simulink model "PLL"  (R2016a)
settings: Solver=ode45  StartTime=0.0  StopTime=stop  MaxStep=1e-6  RelTol=1e-3
values from neighbouring files (symbols this model uses):
  f = 9000    [Aufgabe5.m]
  K0 = 2*pi*400    (= 2513.27412287)    [Aufgabe5.m]
  tau1 = K0*Kd/w0^2    (= 0.000881744837074)    [Aufgabe5.m]
  tau2 = 2*zeta/w0-1/(K0*Kd)    (= 0.000376945917849)    [Aufgabe5.m]
libraries: dspvision x2, dsparch4 x1, commsynccomp2 x1
settings Model: Creator=Martin Buchholz  LastModifiedBy=Marcel
settings DataIOCC: LimitDataPoints=on  SaveFormat=Array  SignalLoggingSaveFormat=ModelDataLogs
settings OptimizationCC: ExpressionDepthLimit=2147483647
settings DebuggingCC: UnderspecifiedInitializationDetection=Classic  MergeDetectMultiDrivingBlocksExec=none  SolverPrmCheckMsg=warning  FcnCallInpInsideContextMsg=UseLocalSettings  StateNameClashWarn=warning
settings HardwareCC: ProdBitPerPointer=32  ProdLargestAtomicFloat=None  ProdIntDivRoundTo=Undefined  ProdEndianess=Unspecified  ProdWordSize=32  ProdHWDeviceType=32-bit Generic
settings ModelReferenceCC: PropagateSignalLabelsOutOfModel=off
settings GRTTargetCC: GeneratePreprocessorConditionals=Use local settings  CombineOutputUpdateFcns=off  GRTInterface=on
settings ConfigComp: CovModelRefEnable=Off

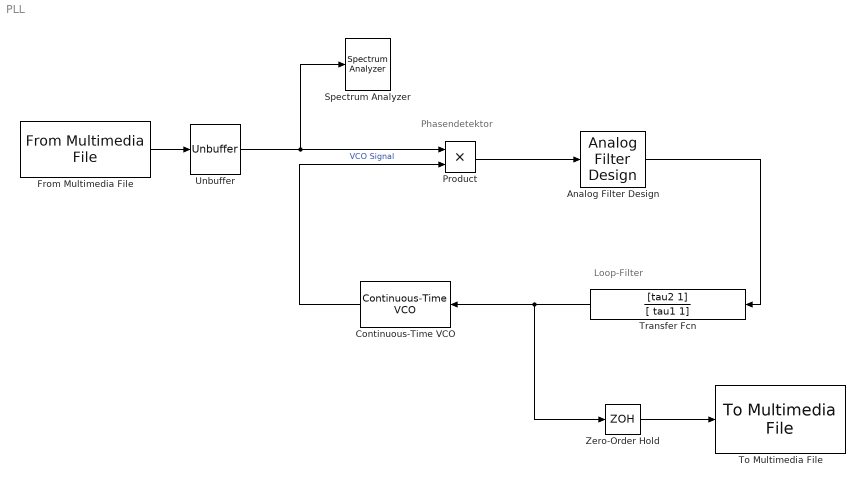
== system PLL ==
  note: Phasendetektor
  note: Loop-Filter
  Analog Filter Design : dsparch4/Analog Filter Design  method=Elliptic  filttype=Lowpass  N=4  Wlo=2*pi*f  Whi=80  Rp=1  Rs=40
  Continuous-Time VCO : commsynccomp2/Continuous-Time VCO  Ac=1  Fc=f  Kc=K0/(2*pi)  Ph=0
  From Multimedia File : dspvision/From Multimedia File  inputFilename=C:\Users\Marcel\Documents\03_GITHUB\Matlab\06_Aufgabe5\Aufgabe5.wav  loop=on  numPlays=1  outputStreams=Audio only  videoDataType=single  audioDataType=double  inheritSampleTime=on  userDefinedSampleTime=1/30  noAudioOutput=off  isIntensityVideo=off  fourcc=RGB  colorVideoFormat=Separate color signals  outputEOF=off  dataOrg=Column-major  audioFrameSize=44100  computeAudioFrameSize=off  outSamplingMode=Sample based
  Product : Product  RndMeth=Zero
  Spectrum Analyzer : SpectrumAnalyzer
  To Multimedia File : dspvision/To Multimedia File  outputFilename=output.wav  streamSelection=Audio only  videoCompressor=None (uncompressed)  audioCompressor=None (uncompressed)  imagePorts=One multidimensional signal  fileType=WAV  audioDatatype=Determine from input data type  fourcc=RGB  videoQuality=75  mj2000CompFactor=10
  Transfer Fcn : TransferFcn  Numerator=[tau2 1]  Denominator=[ tau1 1]
  Unbuffer : Unbuffer  SampleBasedProcessing=Same as frame based
  Zero-Order Hold : ZeroOrderHold  SampleTime=1/44100
  wires:
  Continuous-Time VCO/1 -> Product/2  "VCO Signal"
  Product/1 -> Analog Filter Design/1
  Analog Filter Design/1 -> Transfer Fcn/1
  From Multimedia File/1 -> Unbuffer/1
  Unbuffer/1 -> Spectrum Analyzer/1, Product/1
  Transfer Fcn/1 -> Zero-Order Hold/1, Continuous-Time VCO/1
  Zero-Order Hold/1 -> To Multimedia File/1
